simulink model "model1"  (R2018b)
settings: Solver=VariableStepAuto  StartTime=0.0  StopTime=10.0  RelTol=1e-3
settings Model: Creator=LimeTheCoder  LastModifiedBy=LimeTheCoder

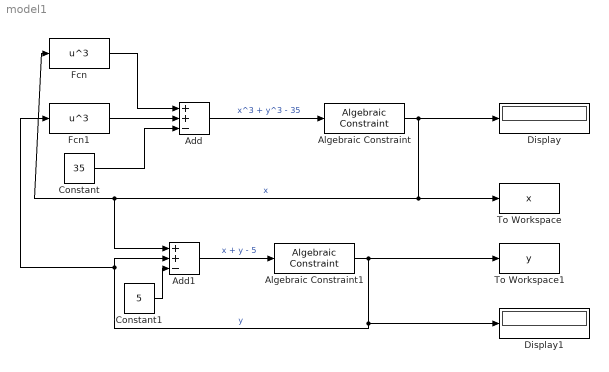
== system model1 ==
  Add : Sum  Inputs=++-
  Add1 : Sum  Inputs=++-
  Algebraic Constraint : AlgebraicConstraint
  Algebraic Constraint1 : AlgebraicConstraint  InitialGuess=1
  Constant : Constant  Value=35
  Constant1 : Constant  Value=5
  Display : Display
  Display1 : Display
  Fcn : Fcn  Expr=u^3
  Fcn1 : Fcn  Expr=u^3
  To Workspace : ToWorkspace  VariableName=x  SampleTime=-1
      settings: MaxDataPoints=1
  To Workspace1 : ToWorkspace  VariableName=y  SampleTime=-1
      settings: MaxDataPoints=1
  wires:
  Fcn/1 -> Add/1
  Fcn1/1 -> Add/2
  Add/1 -> Algebraic Constraint/1  "x^3 + y^3 - 35"
  Algebraic Constraint/1 -> Add1/1, Fcn/1, To Workspace/1, Display/1  "x"
  Algebraic Constraint1/1 -> To Workspace1/1, Add1/2, Fcn1/1, Display1/1  "y"
  Add1/1 -> Algebraic Constraint1/1  "x + y - 5"
  Constant/1 -> Add/3
  Constant1/1 -> Add1/3
